simulink library "Lib_Thermo_SP2T_TMATS"  (R2019b)
settings: Solver=ode45  StartTime=0.0  StopTime=10.0  RelTol=1e-3  EnableMultiTasking=on
Description:
  | Thomas Modules
settings Model: Creator=jwchapm2  LastModifiedBy=bhisma
settings DataIOCC: LimitDataPoints=on  SaveFormat=Array  ReturnWorkspaceOutputs=off
settings OptimizationCC: ExpressionDepthLimit=2147483647  LifeSpan=inf
settings DebuggingCC: UnderspecifiedInitializationDetection=Classic  MergeDetectMultiDrivingBlocksExec=none  SolverPrmCheckMsg=warning  StateNameClashWarn=warning  SFUnexpectedBacktrackingDiag=warning  SFNoUnconditionalDefaultTransitionDiag=warning  SFExecutionAtInitializationDiag=none  ArithmeticOperatorsInVariantConditions=warning
settings HardwareCC: ProdBitPerPointer=32  ProdBitPerSizeT=32  ProdBitPerPtrDiffT=32  ProdLargestAtomicFloat=None  ProdIntDivRoundTo=Undefined  ProdEndianess=Unspecified  ProdWordSize=32  ProdHWDeviceType=32-bit Generic
settings ModelReferenceCC: PropagateSignalLabelsOutOfModel=off
settings SFSimCC: SimUseLocalCustomCode=off  CustomCodeUndefinedFunction=UseInterfaceOnly
settings RTWCC: RTWUseLocalCustomCode=off
settings CodeAppCC: StateflowObjectComments=on
settings GRTTargetCC: TargetLangStandard=C89/C90 (ANSI)  GeneratePreprocessorConditionals=Disable all
settings ConfigComp: CovMetricSettings=dw  CovHtmlReporting=on  CovSaveCumulativeToWorkspaceVar=on  CovSaveSingleToWorkspaceVar=on  CovExternalEMLEnable=off

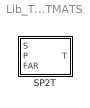
== system Lib_Thermo_SP2T_TMATS ==
  SP2T : Subsystem  mask(T-MATS: SP2T Library Block){}
      mask help: This block emperically calculates temperature (T) from pressure (P), entropy (S) and fuel to air ratio (FAR).
      mask Help: web(which('Thermo_TMATS_SP2T.html'),'-helpbrowser')

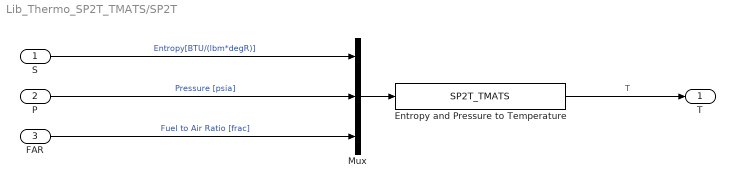
== system Lib_Thermo_SP2T_TMATS/SP2T ==
  S : Inport
  P : Inport  Port=2
  FAR : Inport  Port=3
  Entropy and Pressure to Temperature : S-Function  FunctionName=SP2T_TMATS  SFunctionModules='sp2tc_TMATS'  SFunctionDeploymentMode=off  EnableBusSupport=off
  Mux : Mux  Inputs=3
  T : Outport
  wires:
  Entropy and Pressure to Temperature/1 -> T/1  "T"
  Mux/1 -> Entropy and Pressure to Temperature/1
  S/1 -> Mux/1  "Entropy[BTU/(lbm*degR)]"
  FAR/1 -> Mux/3  "Fuel to Air Ratio [frac]"
  P/1 -> Mux/2  "Pressure [psia]"
